simulink model "FanControl"  (R2018a)
settings: Solver=VariableStepAuto  StartTime=0.0  StopTime=10.0  RelTol=1e-3
settings Model: Creator=Moataz  LastModifiedBy=Moataz

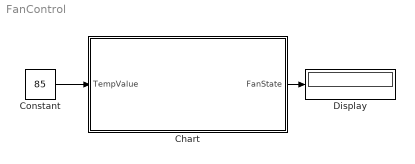
== system FanControl ==
  Chart : Stateflow chart  TreatAsAtomicUnit=on
  Constant : Constant  Value=85  OutDataTypeStr=int8
  Display : Display
  wires:
  Constant/1 -> Chart/1(TempValue)
  Chart/1(FanState) -> Display/1

== stateflow chart FanControl/Chart ==
  note: in case 1: condition action, it is excuted if the condition is TRUE
      | in case 2: transition action , it is excuted if the transition (1&&2) is TRUE
  note: 1
  state FanOFF
    en:  /*Entry*/
    /*Excuted once when you enter the sate*/
    FanState=0;
    du: /*Duration*/
    /*Excuted as long as the SW still in this state */
    ex: /*Exit*/
    /*Excuted once when you leaves the state */
  state FanON
    en:
    FanState=1;
    du:
    ex:
  note: 2
  (default) -> FanOFF : %Default Transition
  FanOFF -> (junction 9) : [TempValue>85]{FANOFFCounter =0;}
  (junction 9) -> FanON : [FanState == ok]/{FANONCounter=10;}
  FanON -> FanOFF : [TempValue<=85]
  data: TempValue input int8 [-55..150]; FanState output boolean [0..1] =0
